simulink model "launcher_simulation"  (R2025b)
settings: Solver=VariableStepAuto  StartTime=0.0  StopTime=5  RelTol=1e-3
values from neighbouring files (symbols this model uses):
  Angle = AngleDegrees * (pi/180)    (= 0.523598775598)    [params.m]    (also in stuff.m = 1.4835298642)
  C_d = 0.5    [params.m]
  C_l = 0.2    [params.m]
  Initial_Height = 0.5    [params.m]    (also in stuff.m = 0)
  omega_val = [0, -5, 0]    [params.m]
  rho = 1.225    [params.m]
  V_mag = 20    [params.m]    (also in stuff.m = v_test_range(i))
settings Model: Creator=Eilon  LastModifiedBy=Eilon

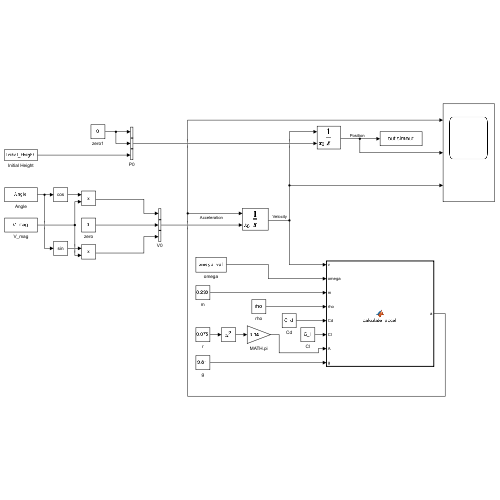
[thumbnail: Simulink's stored preview of the top-level diagram]
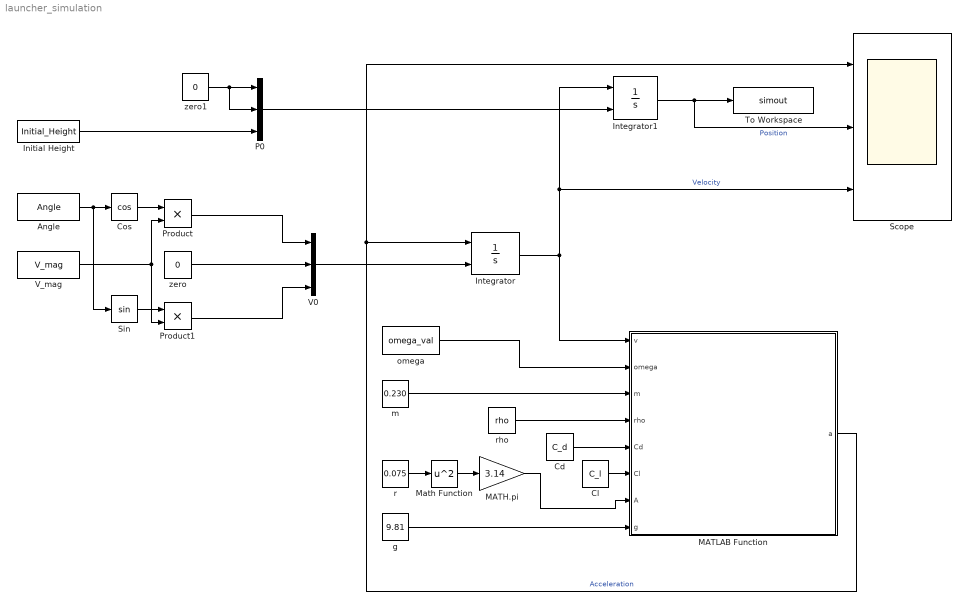
== system launcher_simulation ==
  Angle : Constant  Value=Angle
  Cd : Constant  Value=C_d
  Cl : Constant  Value=C_l
  Cos : Trigonometry  Operator=cos
  Initial Height : Constant  Value=Initial_Height
  Integrator : Integrator  InitialConditionSource=external
  Integrator1 : Integrator  InitialConditionSource=external
  MATH.pi : Gain  Gain=3.14
  MATLAB Function : MATLAB Function  TreatAsAtomicUnit=on
  Math Function : Math  Operator=square
  P0 : Concatenate  NumInputs=3
  Product : Product
  Product1 : Product
  Scope : Scope  NumInputPorts=3
      settings: ActiveDisplayYMinimum=-81.3942383913958  ActiveDisplayYMaximum=122.50735054986983
  Sin : Trigonometry
  To Workspace : ToWorkspace  VariableName=simout  SaveFormat=Timeseries  SampleTime=-1
  V0 : Concatenate  NumInputs=3
  V_mag : Constant  Value=V_mag
  g : Constant  Value=9.81
  m : Constant  Value=0.230
  omega : Constant  Value=omega_val
  r : Constant  Value=0.075
  rho : Constant  Value=rho
  zero : Constant  Value=0
  zero1 : Constant  Value=0
  wires:
  Integrator/1 -> Integrator1/1, Scope/3, MATLAB Function/1(v)  "Velocity"
  MATLAB Function/1(a) -> Integrator/1, Scope/1  "Acceleration"
  Integrator1/1 -> Scope/2, To Workspace/1  "Position"
  g/1 -> MATLAB Function/8(g)
  Math Function/1 -> MATH.pi/1
  MATH.pi/1 -> MATLAB Function/7(A)
  r/1 -> Math Function/1
  m/1 -> MATLAB Function/3(m)
  omega/1 -> MATLAB Function/2(omega)
  Cd/1 -> MATLAB Function/5(Cd)
  Cl/1 -> MATLAB Function/6(Cl)
  rho/1 -> MATLAB Function/4(rho)
  Angle/1 -> Sin/1, Cos/1
  Cos/1 -> Product/1
  Sin/1 -> Product1/1
  V_mag/1 -> Product1/2, Product/2
  Product/1 -> V0/1
  Product1/1 -> V0/3
  zero/1 -> V0/2
  V0/1 -> Integrator/2
  zero1/1 -> P0/2, P0/1
  P0/1 -> Integrator1/2
  Initial Height/1 -> P0/3

== matlab function launcher_simulation/MATLAB Function ==
  data: v input; a output; omega input; m input; rho input; Cd input; Cl input; A input; g input
function a = calculate_accel(v, omega, m, rho, Cd, Cl, A, g)
    % וידוא שכל הוקטורים הם וקטורי עמודה
    v = v(:); 
    omega = omega(:);
    v_mag = norm(v);
    
    % כוחות
    Fg = [0; 0; -m*g]; % כוח כבידה תמיד ב-Z
    Fd = -0.5 * rho * Cd * A * v_mag * v;
    Fm = 0.5 * rho * Cl * A * cross(omega, v); % מכפלה וקטורית יוצרת את ה-3D
    
    a = (Fg + Fd + Fm) / m;
end
